simulink model "BEX3_Speed_Contorl_IncrementalEncoders_BLDC_PMSM_2020a"  (R2021b)
settings: Solver=VariableStepAuto  StartTime=0.0  StopTime=1  RelTol=1e-3
(part 1 of 2)
settings Model: Creator=SL_1  LastModifiedBy=SL_1
settings SolverCC: AlgebraicLoopSolver=TrustRegion

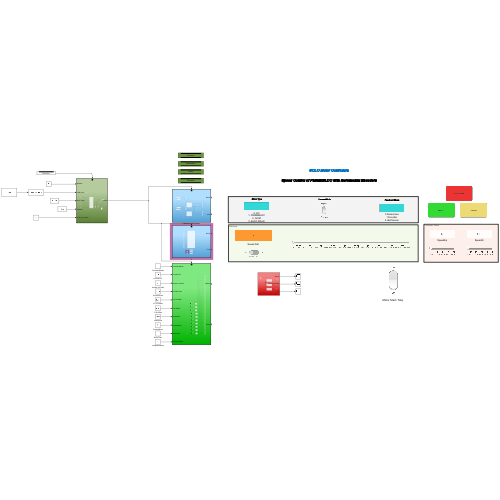
[thumbnail: Simulink's stored preview of the top-level diagram]
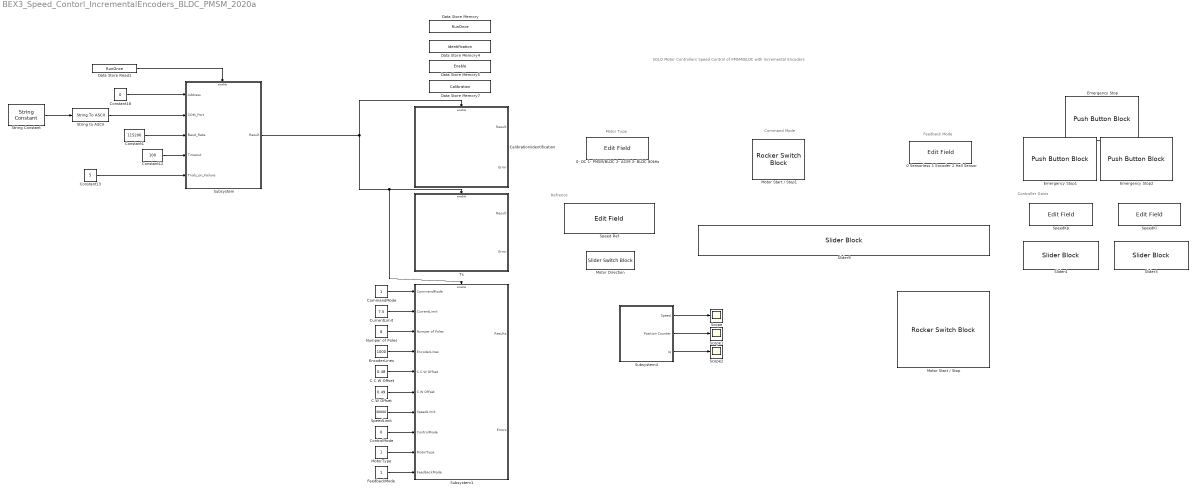
== system BEX3_Speed_Contorl_IncrementalEncoders_BLDC_PMSM_2020a ==
  note: Command Mode
  note: Feedback Mode
  note: Refrence
  note: Controller Gains
  note: SOLO Motor Controllers
      |
      | Speed Control of PMSM/BLDC with Incremental Encoders
  note: Motor Type
  0 Sensorless 1 Encoder 2 Hall Sensor : EditField  LabelPosition=Hide  ShowInitialText=on  Alignment=Center
  "0- DC 1- PMSM/BLDC 2- ACIM 3- BLDC 80kHz " : EditField  LabelPosition=Hide  ShowInitialText=on  Alignment=Center
  C.C.W Offset : Constant  Value=0.48  OutDataTypeStr=single
  C.W Offset : Constant  Value=0.49  OutDataTypeStr=single
  Calibration\Identification : Subsystem
  CommandMode : Constant  OutDataTypeStr=Inherit: Inherit via back propagation  SampleTime=-1
  Constant1 : Constant  Value=115200  OutDataTypeStr=uint32
  Constant12 : Constant  Value=100  OutDataTypeStr=double
  Constant13 : Constant  Value=5  OutDataTypeStr=int32
  Constant18 : Constant  Value=0  OutDataTypeStr=uint8
  ControlMode : Constant  Value=0  OutDataTypeStr=Inherit: Inherit via back propagation
  CurrentLimit : Constant  Value=7.5  OutDataTypeStr=single
  Data Store Memory : DataStoreMemory  DataStoreName=RunOnce  ReadBeforeWriteMsg=warning  WriteAfterWriteMsg=warning  WriteAfterReadMsg=warning  InitialValue=1  ShowAdditionalParam=off  OutDataTypeStr=boolean
  Data Store Memory4 : DataStoreMemory  DataStoreName=Identification  ReadBeforeWriteMsg=warning  WriteAfterWriteMsg=warning  WriteAfterReadMsg=warning  ShowAdditionalParam=off
  Data Store Memory5 : DataStoreMemory  DataStoreName=Enable  ReadBeforeWriteMsg=warning  WriteAfterWriteMsg=warning  WriteAfterReadMsg=warning  ShowAdditionalParam=off
  Data Store Memory7 : DataStoreMemory  DataStoreName=Calibration  ReadBeforeWriteMsg=warning  WriteAfterWriteMsg=warning  WriteAfterReadMsg=warning  ShowAdditionalParam=off
  Data Store Read1 : DataStoreRead  DataStoreName=RunOnce  IndexOptions=Index vector (dialog)  Indices=1  OutputSizes=1
  Emergency Stop : PushButtonBlock  ButtonText=Emergency Stop  OnValue=0  OffValue=1.000000
  Emergency Stop1 : PushButtonBlock  ButtonText=calibration  OffValue=0.000000
  Emergency Stop2 : PushButtonBlock  ButtonText=Identification  OffValue=0.000000
  EncoderLines : Constant  Value=1000  OutDataTypeStr=uint32
  FeedbackMode : Constant  OutDataTypeStr=Inherit: Inherit via back propagation
  Motor Direction : SliderSwitchBlock  LabelPosition=Bottom
      settings: Values={{'CCw', 'Cw'}, [1 0]}
  Motor Start / Stop : RockerSwitchBlock  LabelPosition=Hide
      settings: Values={{'Off', 'On'}, [1 0]}
  Motor Start / Stop1 : RockerSwitchBlock  LabelPosition=Hide
      settings: Values={{'Analog', 'Digital'}, [1 0]}
  MotorType : Constant  OutDataTypeStr=Inherit: Inherit via back propagation
  Numper of Poles : Constant  Value=8  OutDataTypeStr=uint32
  Scope : Scope
  Scope1 : Scope
  Scope2 : Scope
  Slider3 : SliderBlock  LabelPosition=Hide  ScaleMax=5
  Slider4 : SliderBlock  LabelPosition=Hide  ScaleMax=5
  Slider9 : SliderBlock  LabelPosition=Hide  ScaleMax=6000
  Speed Ref : EditField  LabelPosition=Hide  ShowInitialText=on  Alignment=Center
  SpeedKi : EditField  LabelPosition=Hide  ShowInitialText=on  Alignment=Center
  SpeedKp : EditField  LabelPosition=Hide  ShowInitialText=on  Alignment=Center
  SpeedLimit : Constant  Value=30000  OutDataTypeStr=uint32
  String Constant : StringConstant  String="\"COM7\""
  String to ASCII : StringToASCII  OutputVectorSize=5
  Subsystem : Subsystem
  Subsystem1 : Subsystem
  Subsystem4 : Subsystem
  Tx : Subsystem
  wires:
  String Constant/1 -> String to ASCII/1
  Constant18/1 -> Subsystem/1(Address)
  String to ASCII/1 -> Subsystem/2(COM_Port)
  Constant1/1 -> Subsystem/3(Baud_Rate)
  Constant12/1 -> Subsystem/4(Timeout)
  Constant13/1 -> Subsystem/5(Trials_on_Failure)
  FeedbackMode/1 -> Subsystem1/10(FeedbackMode)
  MotorType/1 -> Subsystem1/9(MotorType)
  ControlMode/1 -> Subsystem1/8(ControlMode)
  SpeedLimit/1 -> Subsystem1/7(SpeedLimit)
  C.W Offset/1 -> Subsystem1/6(C.W Offset)
  C.C.W Offset/1 -> Subsystem1/5(C.C.W Offset)
  EncoderLines/1 -> Subsystem1/4(EncoderLines)
  Numper of Poles/1 -> Subsystem1/3(Numper of Poles)
  CurrentLimit/1 -> Subsystem1/2(CurrentLimit)
  CommandMode/1 -> Subsystem1/1(CommandMode)
  Subsystem4/1(Speed) -> Scope/1
  Subsystem4/2(Position Counter) -> Scope1/1
  Subsystem4/3(Iq) -> Scope2/1
  Data Store Read1/1 -> Subsystem/Enable
  Subsystem/1(Result) -> Tx/Enable, Subsystem1/Enable, Calibration\Identification/Enable

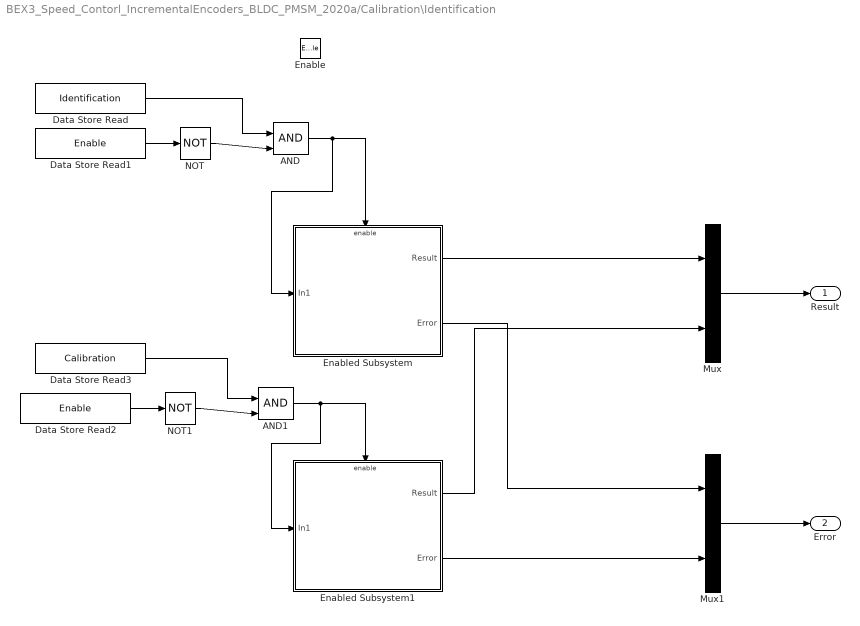
== system BEX3_Speed_Contorl_IncrementalEncoders_BLDC_PMSM_2020a/Calibration\Identification ==
  Enable : EnablePort
  AND : Logic  IconShape=distinctive  AllPortsSameDT=off  OutDataTypeStr=boolean
  AND1 : Logic  IconShape=distinctive  AllPortsSameDT=off  OutDataTypeStr=boolean
  Data Store Read : DataStoreRead  DataStoreName=Identification  IndexOptions=Index vector (dialog)  Indices=1  OutputSizes=1
  Data Store Read1 : DataStoreRead  DataStoreName=Enable  IndexOptions=Index vector (dialog)  Indices=1  OutputSizes=1
  Data Store Read2 : DataStoreRead  DataStoreName=Enable  IndexOptions=Index vector (dialog)  Indices=1  OutputSizes=1
  Data Store Read3 : DataStoreRead  DataStoreName=Calibration  IndexOptions=Index vector (dialog)  Indices=1  OutputSizes=1
  Enabled Subsystem : Subsystem  TreatAsAtomicUnit=on
  Enabled Subsystem1 : Subsystem  TreatAsAtomicUnit=on
  Mux : Mux  Inputs=2
  Mux1 : Mux  Inputs=2
  NOT : Logic  Operator=NOT  IconShape=distinctive  AllPortsSameDT=off  OutDataTypeStr=boolean
  NOT1 : Logic  Operator=NOT  IconShape=distinctive  AllPortsSameDT=off  OutDataTypeStr=boolean
  Result : Outport
  Error : Outport  Port=2
  wires:
  Data Store Read1/1 -> NOT/1
  AND/1 -> Enabled Subsystem/1(In1), Enabled Subsystem/Enable
  NOT/1 -> AND/2
  Data Store Read/1 -> AND/1
  NOT1/1 -> AND1/2
  Data Store Read2/1 -> NOT1/1
  AND1/1 -> Enabled Subsystem1/1(In1), Enabled Subsystem1/Enable
  Data Store Read3/1 -> AND1/1
  Enabled Subsystem/1(Result) -> Mux/1
  Enabled Subsystem/2(Error) -> Mux1/1
  Enabled Subsystem1/2(Error) -> Mux1/2
  Enabled Subsystem1/1(Result) -> Mux/2
  Mux/1 -> Result/1
  Mux1/1 -> Error/1

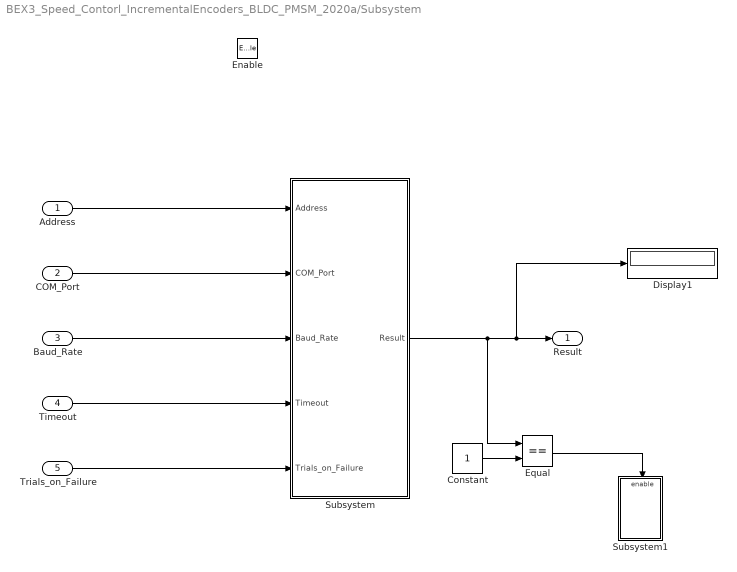
== system BEX3_Speed_Contorl_IncrementalEncoders_BLDC_PMSM_2020a/Subsystem ==
  Address : Inport
  COM_Port : Inport  Port=2
  Baud_Rate : Inport  Port=3
  Timeout : Inport  Port=4
  Trials_on_Failure : Inport  Port=5
  Enable : EnablePort
  Constant : Constant  OutDataTypeStr=Inherit: Inherit via back propagation
  Display1 : Display
  Equal : RelationalOperator  Operator===  OutDataTypeStr=boolean  RndMeth=Simplest
  Subsystem : Subsystem
  Subsystem1 : Subsystem
  Result : Outport
  wires:
  Address/1 -> Subsystem/1(Address)
  COM_Port/1 -> Subsystem/2(COM_Port)
  Baud_Rate/1 -> Subsystem/3(Baud_Rate)
  Timeout/1 -> Subsystem/4(Timeout)
  Trials_on_Failure/1 -> Subsystem/5(Trials_on_Failure)
  Equal/1 -> Subsystem1/Enable
  Subsystem/1(Result) -> Display1/1, Result/1, Equal/1
  Constant/1 -> Equal/2

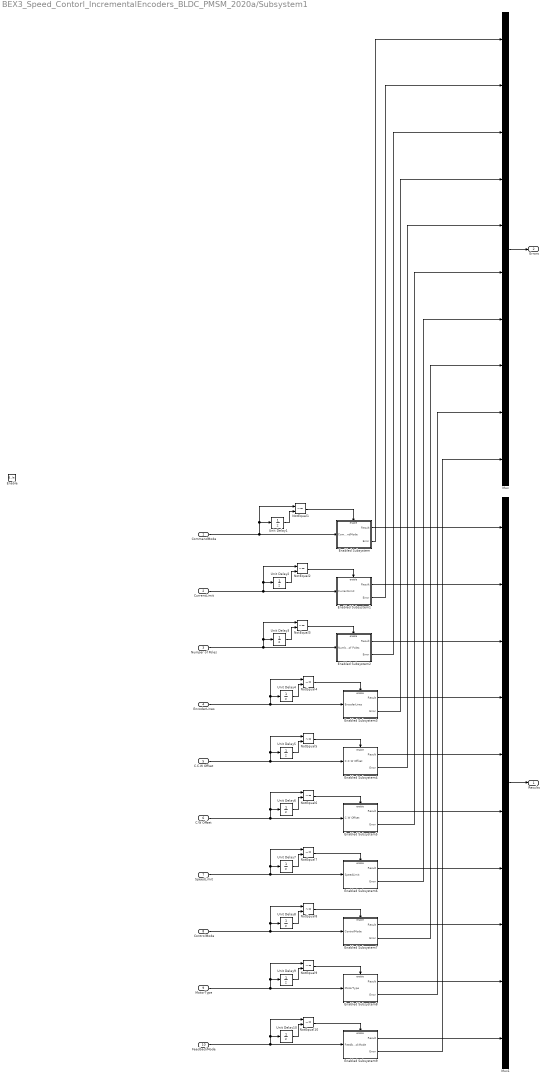
== system BEX3_Speed_Contorl_IncrementalEncoders_BLDC_PMSM_2020a/Subsystem1 ==
  CommandMode : Inport
  CurrentLimit : Inport  Port=2
  Numper of Poles : Inport  Port=3
  EncoderLines : Inport  Port=4
  C.C.W Offset : Inport  Port=5
  C.W Offset : Inport  Port=6
  SpeedLimit : Inport  Port=7
  ControlMode : Inport  Port=8
  MotorType : Inport  Port=9
  FeedbackMode : Inport  Port=10
  Enable : EnablePort
  Enabled Subsystem : Subsystem  TreatAsAtomicUnit=on
  Enabled Subsystem1 : Subsystem  TreatAsAtomicUnit=on
  Enabled Subsystem2 : Subsystem  TreatAsAtomicUnit=on
  Enabled Subsystem3 : Subsystem  TreatAsAtomicUnit=on
  Enabled Subsystem4 : Subsystem  TreatAsAtomicUnit=on
  Enabled Subsystem5 : Subsystem  TreatAsAtomicUnit=on
  Enabled Subsystem6 : Subsystem  TreatAsAtomicUnit=on
  Enabled Subsystem7 : Subsystem  TreatAsAtomicUnit=on
  Enabled Subsystem8 : Subsystem  TreatAsAtomicUnit=on
  Enabled Subsystem9 : Subsystem  TreatAsAtomicUnit=on
  Mux : Mux  Inputs=10
  Mux1 : Mux  Inputs=10
  NotEqual{1..10} (10 alike) : RelationalOperator  Operator=~=  OutDataTypeStr=boolean  RndMeth=Simplest
  Unit Delay{1..10} (10 alike) : UnitDelay  InitialCondition=2.1651  SampleTime=-1  HasFrameUpgradeWarning=on
  Results : Outport
  Errors : Outport  Port=2
  wires:
  Unit Delay1/1 -> NotEqual1/2
  NotEqual1/1 -> Enabled Subsystem/Enable
  NotEqual2/1 -> Enabled Subsystem1/Enable
  CurrentLimit/1 -> NotEqual2/1, Unit Delay2/1, Enabled Subsystem1/1(CurrentLimit)
  Unit Delay2/1 -> NotEqual2/2
  Unit Delay3/1 -> NotEqual3/2
  Numper of Poles/1 -> Enabled Subsystem2/1(Number of Poles), Unit Delay3/1, NotEqual3/1
  NotEqual3/1 -> Enabled Subsystem2/Enable
  NotEqual4/1 -> Enabled Subsystem3/Enable
  EncoderLines/1 -> NotEqual4/1, Unit Delay4/1, Enabled Subsystem3/1(EncoderLines)
  Unit Delay4/1 -> NotEqual4/2
  Unit Delay5/1 -> NotEqual5/2
  C.C.W Offset/1 -> Enabled Subsystem4/1(C.C.W Offset), Unit Delay5/1, NotEqual5/1
  NotEqual5/1 -> Enabled Subsystem4/Enable
  NotEqual6/1 -> Enabled Subsystem5/Enable
  C.W Offset/1 -> NotEqual6/1, Unit Delay6/1, Enabled Subsystem5/1(C.W Offset)
  Unit Delay6/1 -> NotEqual6/2
  Unit Delay7/1 -> NotEqual7/2
  SpeedLimit/1 -> Enabled Subsystem6/1(SpeedLimit), Unit Delay7/1, NotEqual7/1
  NotEqual7/1 -> Enabled Subsystem6/Enable
  NotEqual8/1 -> Enabled Subsystem7/Enable
  ControlMode/1 -> NotEqual8/1, Unit Delay8/1, Enabled Subsystem7/1(ControlMode)
  Unit Delay8/1 -> NotEqual8/2
  Unit Delay9/1 -> NotEqual9/2
  MotorType/1 -> Enabled Subsystem8/1(MotorType), Unit Delay9/1, NotEqual9/1
  NotEqual9/1 -> Enabled Subsystem8/Enable
  NotEqual10/1 -> Enabled Subsystem9/Enable
  FeedbackMode/1 -> NotEqual10/1, Unit Delay10/1, Enabled Subsystem9/1(FeedbackMode)
  Unit Delay10/1 -> NotEqual10/2
  CommandMode/1 -> Enabled Subsystem/1(CommandMode), NotEqual1/1, Unit Delay1/1
  Enabled Subsystem9/2(Error) -> Mux/10
  Enabled Subsystem8/2(Error) -> Mux/9
  Enabled Subsystem7/2(Error) -> Mux/8
  Enabled Subsystem6/2(Error) -> Mux/7
  Enabled Subsystem5/2(Error) -> Mux/6
  Enabled Subsystem4/2(Error) -> Mux/5
  Enabled Subsystem3/2(Error) -> Mux/4
  Enabled Subsystem2/2(Error) -> Mux/3
  Enabled Subsystem1/2(Error) -> Mux/2
  Enabled Subsystem/2(Error) -> Mux/1
  Enabled Subsystem/1(Result) -> Mux1/1
  Enabled Subsystem1/1(Result) -> Mux1/2
  Enabled Subsystem2/1(Result) -> Mux1/3
  Enabled Subsystem3/1(Result) -> Mux1/4
  Enabled Subsystem5/1(Result) -> Mux1/6
  Enabled Subsystem7/1(Result) -> Mux1/8
  Enabled Subsystem6/1(Result) -> Mux1/7
  Enabled Subsystem8/1(Result) -> Mux1/9
  Enabled Subsystem9/1(Result) -> Mux1/10
  Enabled Subsystem4/1(Result) -> Mux1/5
  Mux1/1 -> Results/1
  Mux/1 -> Errors/1

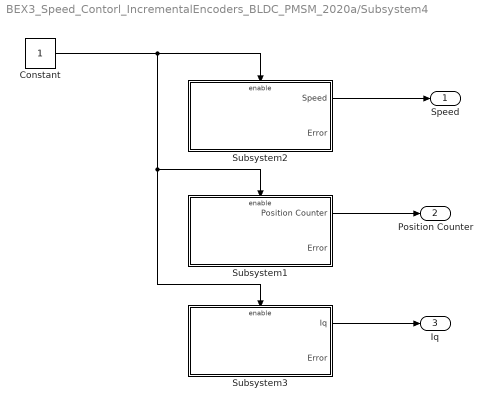
== system BEX3_Speed_Contorl_IncrementalEncoders_BLDC_PMSM_2020a/Subsystem4 ==
  Constant : Constant  SampleTime=1e-3
  Subsystem1 : Subsystem
  Subsystem2 : Subsystem
  Subsystem3 : Subsystem
  Speed : Outport
  Position Counter : Outport  Port=2
  Iq : Outport  Port=3
  wires:
  Constant/1 -> Subsystem1/Enable, Subsystem3/Enable, Subsystem2/Enable
  Subsystem2/1(Speed) -> Speed/1
  Subsystem1/1(Position Counter) -> Position Counter/1
  Subsystem3/1(Iq) -> Iq/1

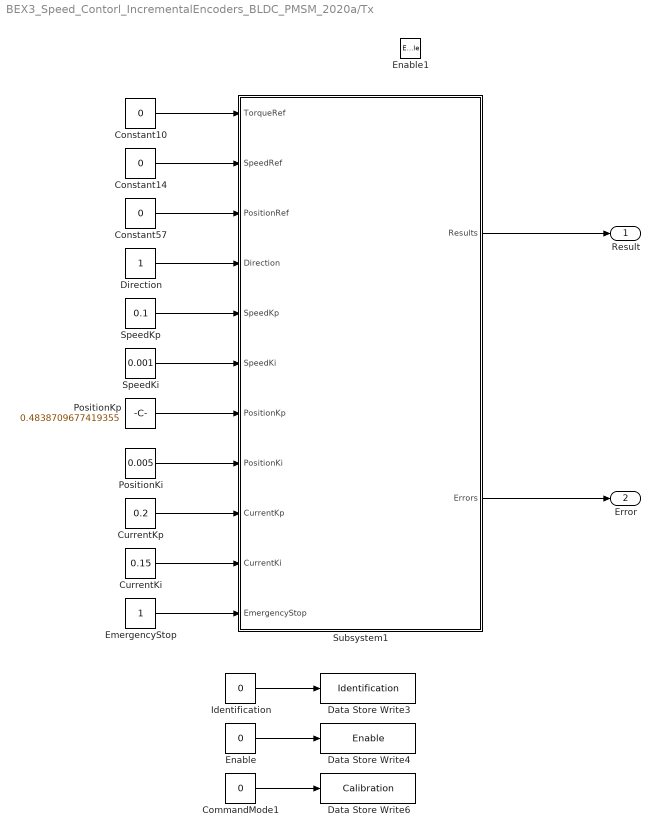
== system BEX3_Speed_Contorl_IncrementalEncoders_BLDC_PMSM_2020a/Tx ==
  Enable1 : EnablePort
  CommandMode1 : Constant  Value=0  OutDataTypeStr=Inherit: Inherit via back propagation
  Constant10 : Constant  Value=0  OutDataTypeStr=Inherit: Inherit via back propagation
  Constant14 : Constant  Value=0  OutDataTypeStr=Inherit: Inherit via back propagation
  Constant57 : Constant  Value=0  OutDataTypeStr=Inherit: Inherit via back propagation
  CurrentKi : Constant  Value=0.15  OutDataTypeStr=Inherit: Inherit via back propagation
  CurrentKp : Constant  Value=0.2  OutDataTypeStr=Inherit: Inherit via back propagation
  Data Store Write3 : DataStoreWrite  DataStoreName=Identification  IndexOptions=Index vector (dialog)  Indices=1  OutputSizes=1
  Data Store Write4 : DataStoreWrite  DataStoreName=Enable  IndexOptions=Index vector (dialog)  Indices=1  OutputSizes=1
  Data Store Write6 : DataStoreWrite  DataStoreName=Calibration  IndexOptions=Index vector (dialog)  Indices=1  OutputSizes=1
  Direction : Constant  OutDataTypeStr=Inherit: Inherit via back propagation
  EmergencyStop : Constant  OutDataTypeStr=boolean
  Enable : Constant  Value=0  OutDataTypeStr=Inherit: Inherit via back propagation
  Identification : Constant  Value=0  OutDataTypeStr=Inherit: Inherit via back propagation
  PositionKi : Constant  Value=0.005  OutDataTypeStr=Inherit: Inherit via back propagation
  PositionKp : Constant  Value=0.4838709677419355  OutDataTypeStr=Inherit: Inherit via back propagation
  SpeedKi : Constant  Value=0.001  OutDataTypeStr=Inherit: Inherit via back propagation
  SpeedKp : Constant  Value=0.1  OutDataTypeStr=Inherit: Inherit via back propagation
  Subsystem1 : Subsystem
  Result : Outport
  Error : Outport  Port=2
  wires:
  Direction/1 -> Subsystem1/4(Direction)
  Constant10/1 -> Subsystem1/1(TorqueRef)
  Constant14/1 -> Subsystem1/2(SpeedRef)
  Constant57/1 -> Subsystem1/3(PositionRef)
  CurrentKi/1 -> Subsystem1/10(CurrentKi)
  CurrentKp/1 -> Subsystem1/9(CurrentKp)
  PositionKi/1 -> Subsystem1/8(PositionKi)
  PositionKp/1 -> Subsystem1/7(PositionKp)
  SpeedKi/1 -> Subsystem1/6(SpeedKi)
  SpeedKp/1 -> Subsystem1/5(SpeedKp)
  Identification/1 -> Data Store Write3/1
  Enable/1 -> Data Store Write4/1
  EmergencyStop/1 -> Subsystem1/11(EmergencyStop)
  CommandMode1/1 -> Data Store Write6/1
  Subsystem1/1(Results) -> Result/1
  Subsystem1/2(Errors) -> Error/1

== system BEX3_Speed_Contorl_IncrementalEncoders_BLDC_PMSM_2020a/Calibration\Identification/Enabled Subsystem ==
  In1 : Inport
  Enable : EnablePort
  Constant21 : Constant  Value=0  OutDataTypeStr=uint8
  MotorParameterIdentification : Subsystem
  Result : Outport
  Error : Outport  Port=2
  wires:
  In1/1 -> MotorParameterIdentification/2(Value)
  Constant21/1 -> MotorParameterIdentification/1(Address)
  MotorParameterIdentification/1(Result) -> Result/1
  MotorParameterIdentification/2(Error) -> Error/1

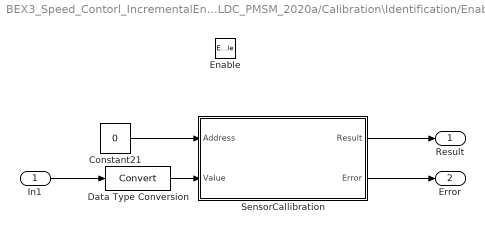
== system BEX3_Speed_Contorl_IncrementalEncoders_BLDC_PMSM_2020a/Calibration\Identification/Enabled Subsystem1 ==
  In1 : Inport
  Enable : EnablePort
  Constant21 : Constant  Value=0  OutDataTypeStr=uint8
  Data Type Conversion : DataTypeConversion
  SensorCallibration : Subsystem
  Result : Outport
  Error : Outport  Port=2
  wires:
  Constant21/1 -> SensorCallibration/1(Address)
  In1/1 -> Data Type Conversion/1
  Data Type Conversion/1 -> SensorCallibration/2(Value)
  SensorCallibration/1(Result) -> Result/1
  SensorCallibration/2(Error) -> Error/1

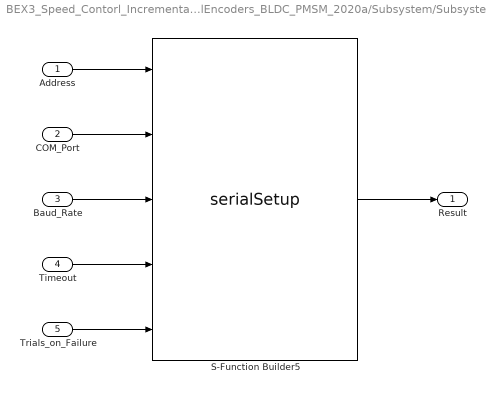
== system BEX3_Speed_Contorl_IncrementalEncoders_BLDC_PMSM_2020a/Subsystem/Subsystem ==
  Address : Inport
  COM_Port : Inport  Port=2
  Baud_Rate : Inport  Port=3
  Timeout : Inport  Port=4
  Trials_on_Failure : Inport  Port=5
  S-Function Builder5 : S-Function  Priority=1  FunctionName=serialSetup  SFunctionModules=serialSetup_wrapper  SFunctionDeploymentMode=off  EnableBusSupport=off  mask(S-Function Builder){}
      mask help: Simulink:masks:SFunctionBuilder_MD
      mask init:
      | val = [[.9  0.75 0.75 1 1 .9 .9 1]',[1 1 0.75 0.75 .9 .9 1 .9]'];try , sys = get_param(gcb,'SfunBuilderFcnName');if isempty(sys), sys = get_param(gcb,'FunctionName'); end,catch, sys = get_param(gcb,'FunctionName'); end
      settings: CopyFcn=set_param(gcbh,'LinkStatus','none')  OpenFcn=sfunctionwizard(gcbh)
      mask Display: plot(val(:,1),val(:,2)),disp(sys),port_label('input',1,'Address'),port_label('input',2,'COM_Port'),port_label('input',3,'Baud_Rate'),port_label('input',4,'Timeout'),port_label('input',5,'Trials_on_Failure'),port_label('output',1,'Result')
  Result : Outport
  wires:
  S-Function Builder5/1 -> Result/1
  COM_Port/1 -> S-Function Builder5/2
  Address/1 -> S-Function Builder5/1
  Timeout/1 -> S-Function Builder5/4
  Baud_Rate/1 -> S-Function Builder5/3
  Trials_on_Failure/1 -> S-Function Builder5/5

== system BEX3_Speed_Contorl_IncrementalEncoders_BLDC_PMSM_2020a/Subsystem/Subsystem1 ==
  Enable : EnablePort
  Constant1 : Constant  Value=0  OutDataTypeStr=Inherit: Inherit via back propagation
  Data Store Write : DataStoreWrite  DataStoreName=RunOnce  IndexOptions=Index vector (dialog)  Indices=1  OutputSizes=1
  wires:
  Constant1/1 -> Data Store Write/1

== system BEX3_Speed_Contorl_IncrementalEncoders_BLDC_PMSM_2020a/Subsystem1/Enabled Subsystem ==
  CommandMode : Inport
  Enable : EnablePort
  Constant6 : Constant  Value=0  OutDataTypeStr=Inherit: Inherit via back propagation
  SetCommandMode : Subsystem
  Result : Outport
  Error : Outport  Port=2
  wires:
  Constant6/1 -> SetCommandMode/1(Address)
  CommandMode/1 -> SetCommandMode/2(Value)
  SetCommandMode/1(Result) -> Result/1
  SetCommandMode/2(Error) -> Error/1

== system BEX3_Speed_Contorl_IncrementalEncoders_BLDC_PMSM_2020a/Subsystem1/Enabled Subsystem1 ==
  CurrentLimit : Inport
  Enable : EnablePort
  Constant6 : Constant  Value=0  OutDataTypeStr=uint8
  SetCurrentLimit : Subsystem
  Result : Outport
  Error : Outport  Port=2
  wires:
  Constant6/1 -> SetCurrentLimit/1(Address)
  CurrentLimit/1 -> SetCurrentLimit/2(Value)
  SetCurrentLimit/2(Error) -> Error/1
  SetCurrentLimit/1(Result) -> Result/1

== system BEX3_Speed_Contorl_IncrementalEncoders_BLDC_PMSM_2020a/Subsystem1/Enabled Subsystem2 ==
  Number of Poles : Inport
  Enable : EnablePort
  Constant6 : Constant  Value=0  OutDataTypeStr=uint8
  SetMotorPoleCounts : Subsystem
  Result : Outport
  Error : Outport  Port=2
  wires:
  Number of Poles/1 -> SetMotorPoleCounts/2(Value)
  Constant6/1 -> SetMotorPoleCounts/1(Address)
  SetMotorPoleCounts/2(Error) -> Error/1
  SetMotorPoleCounts/1(Result) -> Result/1

== system BEX3_Speed_Contorl_IncrementalEncoders_BLDC_PMSM_2020a/Subsystem1/Enabled Subsystem3 ==
  EncoderLines : Inport
  Enable : EnablePort
  Constant6 : Constant  Value=0  OutDataTypeStr=uint8
  SetEncoderLines : Subsystem
  Result : Outport
  Error : Outport  Port=2
  wires:
  Constant6/1 -> SetEncoderLines/1(Address)
  EncoderLines/1 -> SetEncoderLines/2(Value)
  SetEncoderLines/2(Error) -> Error/1
  SetEncoderLines/1(Result) -> Result/1

== system BEX3_Speed_Contorl_IncrementalEncoders_BLDC_PMSM_2020a/Subsystem1/Enabled Subsystem4 ==
  C.C.W Offset : Inport
  Enable : EnablePort
  Constant6 : Constant  Value=0  OutDataTypeStr=uint8
  SetEncoderHallCcwOffset : Subsystem
  Result : Outport
  Error : Outport  Port=2
  wires:
  C.C.W Offset/1 -> SetEncoderHallCcwOffset/2(Value)
  Constant6/1 -> SetEncoderHallCcwOffset/1(Address)
  SetEncoderHallCcwOffset/2(Error) -> Error/1
  SetEncoderHallCcwOffset/1(Result) -> Result/1

== system BEX3_Speed_Contorl_IncrementalEncoders_BLDC_PMSM_2020a/Subsystem1/Enabled Subsystem5 ==
  C.W Offset : Inport
  Enable : EnablePort
  Constant6 : Constant  Value=0  OutDataTypeStr=uint8
  SetEncoderHallCwOffset : Subsystem
  Result : Outport
  Error : Outport  Port=2
  wires:
  Constant6/1 -> SetEncoderHallCwOffset/1(Address)
  C.W Offset/1 -> SetEncoderHallCwOffset/2(Value)
  SetEncoderHallCwOffset/2(Error) -> Error/1
  SetEncoderHallCwOffset/1(Result) -> Result/1

== system BEX3_Speed_Contorl_IncrementalEncoders_BLDC_PMSM_2020a/Subsystem1/Enabled Subsystem6 ==
  SpeedLimit : Inport
  Enable : EnablePort
  Constant6 : Constant  Value=0  OutDataTypeStr=uint8
  SetSpeedLimit : Subsystem
  Result : Outport
  Error : Outport  Port=2
  wires:
  SpeedLimit/1 -> SetSpeedLimit/2(Value)
  Constant6/1 -> SetSpeedLimit/1(Address)
  SetSpeedLimit/2(Error) -> Error/1
  SetSpeedLimit/1(Result) -> Result/1

== system BEX3_Speed_Contorl_IncrementalEncoders_BLDC_PMSM_2020a/Subsystem1/Enabled Subsystem7 ==
  ControlMode : Inport
  Enable : EnablePort
  Constant6 : Constant  Value=0  OutDataTypeStr=uint8
  SetControlMode : Subsystem
  Result : Outport
  Error : Outport  Port=2
  wires:
  Constant6/1 -> SetControlMode/1(Address)
  ControlMode/1 -> SetControlMode/2(Value)
  SetControlMode/2(Error) -> Error/1
  SetControlMode/1(Result) -> Result/1

== system BEX3_Speed_Contorl_IncrementalEncoders_BLDC_PMSM_2020a/Subsystem1/Enabled Subsystem8 ==
  MotorType : Inport
  Enable : EnablePort
  Constant6 : Constant  Value=0  OutDataTypeStr=uint8
  SetMotorType : Subsystem
  Result : Outport
  Error : Outport  Port=2
  wires:
  MotorType/1 -> SetMotorType/2(Value)
  Constant6/1 -> SetMotorType/1(Address)
  SetMotorType/2(Error) -> Error/1
  SetMotorType/1(Result) -> Result/1

== system BEX3_Speed_Contorl_IncrementalEncoders_BLDC_PMSM_2020a/Subsystem1/Enabled Subsystem9 ==
  FeedbackMode : Inport
  Enable : EnablePort
  Constant6 : Constant  Value=0  OutDataTypeStr=uint8
  SetFeedBackControlMode : Subsystem
  Result : Outport
  Error : Outport  Port=2
  wires:
  Constant6/1 -> SetFeedBackControlMode/1(Address)
  FeedbackMode/1 -> SetFeedBackControlMode/2(Value)
  SetFeedBackControlMode/2(Error) -> Error/1
  SetFeedBackControlMode/1(Result) -> Result/1

== system BEX3_Speed_Contorl_IncrementalEncoders_BLDC_PMSM_2020a/Subsystem4/Subsystem1 ==
  Enable : EnablePort
  Constant120 : Constant  Value=0  OutDataTypeStr=uint8
  GetPositionCountsFeedback : Subsystem
  Position Counter : Outport
  Error : Outport  Port=2
  wires:
  Constant120/1 -> GetPositionCountsFeedback/1(Address)
  GetPositionCountsFeedback/1(Result) -> Position Counter/1
  GetPositionCountsFeedback/2(Error) -> Error/1

== system BEX3_Speed_Contorl_IncrementalEncoders_BLDC_PMSM_2020a/Subsystem4/Subsystem2 ==
  Enable : EnablePort
  Constant120 : Constant  Value=0  OutDataTypeStr=uint8
  GetSpeedFeedback : Subsystem
  Speed : Outport
  Error : Outport  Port=2
  wires:
  GetSpeedFeedback/1(Result) -> Speed/1
  Constant120/1 -> GetSpeedFeedback/1(Address)
  GetSpeedFeedback/2(Error) -> Error/1

== system BEX3_Speed_Contorl_IncrementalEncoders_BLDC_PMSM_2020a/Subsystem4/Subsystem3 ==
  Enable : EnablePort
  Constant120 : Constant  Value=0  OutDataTypeStr=uint8
  GetQuadratureCurrentIqFeedback : Subsystem
  Iq : Outport
  Error : Outport  Port=2
  wires:
  GetQuadratureCurrentIqFeedback/2(Error) -> Error/1
  GetQuadratureCurrentIqFeedback/1(Result) -> Iq/1
  Constant120/1 -> GetQuadratureCurrentIqFeedback/1(Address)

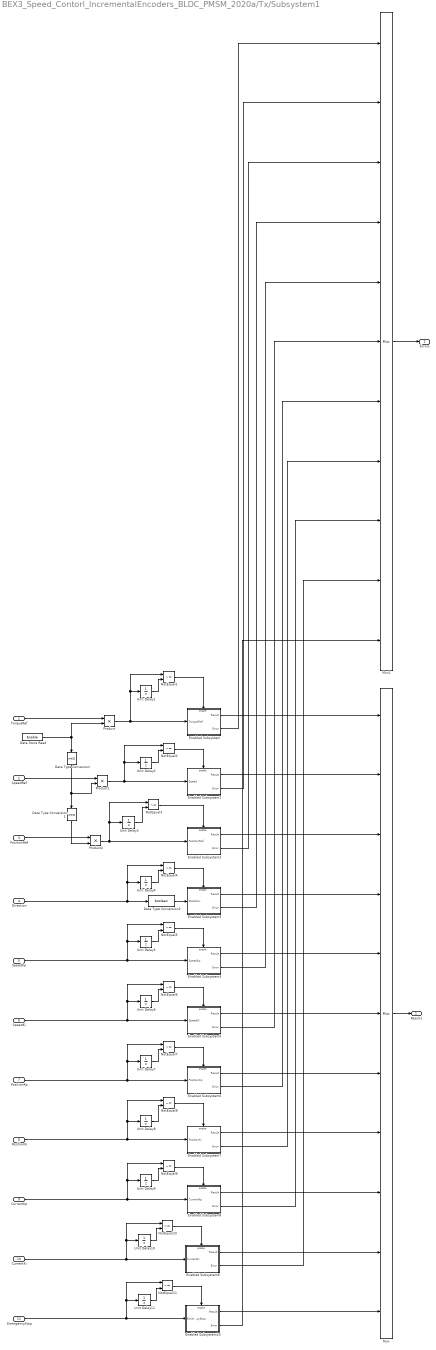
== system BEX3_Speed_Contorl_IncrementalEncoders_BLDC_PMSM_2020a/Tx/Subsystem1 ==
  TorqueRef : Inport
  SpeedRef : Inport  Port=2
  PositionRef : Inport  Port=3
  Direction : Inport  Port=4
  SpeedKp : Inport  Port=5
  SpeedKi : Inport  Port=6
  PositionKp : Inport  Port=7
  PositionKi : Inport  Port=8
  CurrentKp : Inport  Port=9
  CurrentKi : Inport  Port=10
  EmergencyStop : Inport  Port=11
  Data Store Read : DataStoreRead  DataStoreName=Enable  IndexOptions=Index vector (dialog)  Indices=1  OutputSizes=1
  Data Type Conversion : DataTypeConversion  OutDataTypeStr=uint32
  Data Type Conversion1 : DataTypeConversion  OutDataTypeStr=uint32
  Data Type Conversion2 : DataTypeConversion  OutDataTypeStr=boolean
  Enabled Subsystem : Subsystem  TreatAsAtomicUnit=on
  Enabled Subsystem1 : Subsystem  TreatAsAtomicUnit=on
  Enabled Subsystem10 : Subsystem  TreatAsAtomicUnit=on
  Enabled Subsystem2 : Subsystem  TreatAsAtomicUnit=on
  Enabled Subsystem3 : Subsystem  TreatAsAtomicUnit=on
  Enabled Subsystem4 : Subsystem  TreatAsAtomicUnit=on
  Enabled Subsystem5 : Subsystem  TreatAsAtomicUnit=on
  Enabled Subsystem6 : Subsystem  TreatAsAtomicUnit=on
  Enabled Subsystem7 : Subsystem  TreatAsAtomicUnit=on
  Enabled Subsystem8 : Subsystem  TreatAsAtomicUnit=on
  Enabled Subsystem9 : Subsystem  TreatAsAtomicUnit=on
  Mux : Mux  Inputs=11
  Mux1 : Mux  Inputs=11
  NotEqual{1..11} (11 alike) : RelationalOperator  Operator=~=  OutDataTypeStr=boolean  RndMeth=Simplest
  Product : Product
  Product1 : Product  OutDataTypeStr=Inherit: Inherit via back propagation
  Product2 : Product  OutDataTypeStr=Inherit: Inherit via back propagation
  Unit Delay{1..11} (11 alike) : UnitDelay  InitialCondition=2.1651  SampleTime=-1  HasFrameUpgradeWarning=on
  Results : Outport
  Errors : Outport  Port=2
  wires:
  TorqueRef/1 -> Product/1
  Unit Delay1/1 -> NotEqual1/2
  NotEqual1/1 -> Enabled Subsystem/Enable
  Data Store Read/1 -> Data Type Conversion/1, Product/2
  Product/1 -> Enabled Subsystem/1(TorqueRef), Unit Delay1/1, NotEqual1/1
  NotEqual2/1 -> Enabled Subsystem1/Enable
  Unit Delay2/1 -> NotEqual2/2
  SpeedRef/1 -> Product1/1
  Product1/1 -> Unit Delay2/1, NotEqual2/1, Enabled Subsystem1/1(Speed)
  PositionRef/1 -> Product2/1
  Unit Delay3/1 -> NotEqual3/2
  NotEqual3/1 -> Enabled Subsystem2/Enable
  Direction/1 -> NotEqual4/1, Unit Delay4/1, Data Type Conversion2/1
  Unit Delay4/1 -> NotEqual4/2
  NotEqual4/1 -> Enabled Subsystem3/Enable
  NotEqual5/1 -> Enabled Subsystem4/Enable
  Unit Delay5/1 -> NotEqual5/2
  SpeedKp/1 -> Enabled Subsystem4/1(SpeedKp), Unit Delay5/1, NotEqual5/1
  SpeedKi/1 -> Enabled Subsystem5/1(SpeedKi), NotEqual6/1, Unit Delay6/1
  Unit Delay6/1 -> NotEqual6/2
  NotEqual6/1 -> Enabled Subsystem5/Enable
  NotEqual7/1 -> Enabled Subsystem6/Enable
  Unit Delay7/1 -> NotEqual7/2
  PositionKp/1 -> Enabled Subsystem6/1(PositionKp), Unit Delay7/1, NotEqual7/1
  PositionKi/1 -> Enabled Subsystem7/1(PositionKi), NotEqual8/1, Unit Delay8/1
  Unit Delay8/1 -> NotEqual8/2
  NotEqual8/1 -> Enabled Subsystem7/Enable
  NotEqual9/1 -> Enabled Subsystem8/Enable
  Unit Delay9/1 -> NotEqual9/2
  CurrentKp/1 -> Enabled Subsystem8/1(CurrentKp), Unit Delay9/1, NotEqual9/1
  CurrentKi/1 -> Enabled Subsystem9/1(CurrentKi), NotEqual10/1, Unit Delay10/1
  Unit Delay10/1 -> NotEqual10/2
  NotEqual10/1 -> Enabled Subsystem9/Enable
  NotEqual11/1 -> Enabled Subsystem10/Enable
  Unit Delay11/1 -> NotEqual11/2
  EmergencyStop/1 -> Unit Delay11/1, NotEqual11/1, Enabled Subsystem10/1(EmergencyStop)
  Data Type Conversion/1 -> Product1/2, Data Type Conversion1/1
  Data Type Conversion1/1 -> Product2/2
  Product2/1 -> NotEqual3/1, Unit Delay3/1, Enabled Subsystem2/1(PositionRef)
  Data Type Conversion2/1 -> Enabled Subsystem3/1(Direction)
  Enabled Subsystem/1(Result) -> Mux/1
  Enabled Subsystem10/1(Result) -> Mux/11
  Enabled Subsystem9/1(Result) -> Mux/10
  Enabled Subsystem8/1(Result) -> Mux/9
  Enabled Subsystem7/1(Result) -> Mux/8
  Enabled Subsystem6/1(Result) -> Mux/7
  Enabled Subsystem5/1(Result) -> Mux/6
  Enabled Subsystem4/1(Result) -> Mux/5
  Enabled Subsystem3/1(Result) -> Mux/4
  Enabled Subsystem2/1(Result) -> Mux/3
  Enabled Subsystem1/1(Result) -> Mux/2
  Mux/1 -> Results/1
  Enabled Subsystem/2(Error) -> Mux1/1
  Enabled Subsystem1/2(Error) -> Mux1/2
  Enabled Subsystem2/2(Error) -> Mux1/3
  Enabled Subsystem3/2(Error) -> Mux1/4
  Enabled Subsystem4/2(Error) -> Mux1/5
  Enabled Subsystem5/2(Error) -> Mux1/6
  Enabled Subsystem6/2(Error) -> Mux1/7
  Enabled Subsystem7/2(Error) -> Mux1/8
  Enabled Subsystem8/2(Error) -> Mux1/9
  Enabled Subsystem9/2(Error) -> Mux1/10
  Enabled Subsystem10/2(Error) -> Mux1/11
  Mux1/1 -> Errors/1

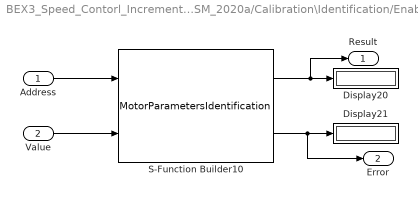
== system BEX3_Speed_Contorl_IncrementalEncoders_BLDC_PMSM_2020a/Calibration\Identification/Enabled Subsystem/MotorParameterIdentification ==
  Address : Inport
  Value : Inport  Port=2
  Display20 : Display
      settings: Format=decimal (Stored Integer)
  Display21 : Display
      settings: Format=decimal (Stored Integer)
  S-Function Builder10 : S-Function  Priority=2  FunctionName=MotorParametersIdentification  SFunctionModules=MotorParametersIdentification_wrapper  SFunctionDeploymentMode=off  EnableBusSupport=off  mask(S-Function Builder){}
      mask help: Simulink:masks:SFunctionBuilder_MD
      mask init: same as BEX3_Speed_Contorl_IncrementalEncoders_BLDC_PMSM_2020a/Subsystem/Subsystem/S-Function Builder5
      settings: CopyFcn=set_param(gcbh,'LinkStatus','none')  OpenFcn=sfunctionwizard(gcbh)
      mask Display:
      | plot(val(:,1),val(:,2))
      | disp(sys)
      | port_label('input',1,'Address')
      | port_label('input',2,'Value')
      | port_label('output',1,'Result')
      | port_label('output',2,'Error')
  Result : Outport
  Error : Outport  Port=2
  wires:
  S-Function Builder10/2 -> Error/1, Display21/1
  S-Function Builder10/1 -> Result/1, Display20/1
  Value/1 -> S-Function Builder10/2
  Address/1 -> S-Function Builder10/1

== system BEX3_Speed_Contorl_IncrementalEncoders_BLDC_PMSM_2020a/Calibration\Identification/Enabled Subsystem1/SensorCallibration ==
  Address : Inport
  Value : Inport  Port=2
  S-Function Builder41 : S-Function  Priority=2  FunctionName=SensorCalibration  SFunctionModules=SensorCalibration_wrapper  SFunctionDeploymentMode=off  EnableBusSupport=off  mask(S-Function Builder){}
      mask help: Simulink:masks:SFunctionBuilder_MD
      mask init: same as BEX3_Speed_Contorl_IncrementalEncoders_BLDC_PMSM_2020a/Subsystem/Subsystem/S-Function Builder5
      settings: CopyFcn=set_param(gcbh,'LinkStatus','none')  OpenFcn=sfunctionwizard(gcbh)
      mask Display:
      | plot(val(:,1),val(:,2))
      | disp(sys)
      | port_label('input',1,'Address')
      | port_label('input',2,'Value')
      | port_label('output',1,'Result')
      | port_label('output',2,'Error')
  Result : Outport
  Error : Outport  Port=2
  wires:
  Value/1 -> S-Function Builder41/2
  S-Function Builder41/1 -> Result/1
  Address/1 -> S-Function Builder41/1
  S-Function Builder41/2 -> Error/1

== system BEX3_Speed_Contorl_IncrementalEncoders_BLDC_PMSM_2020a/Subsystem1/Enabled Subsystem/SetCommandMode ==
  Address : Inport  OutDataTypeStr=uint8  LockScale=on
  Value : Inport  Port=2  OutDataTypeStr=boolean  LockScale=on
  S-Function Builder2 : S-Function  Priority=2  FunctionName=SetCommandMode  SFunctionModules=SetCommandMode_wrapper  SFunctionDeploymentMode=off  EnableBusSupport=off  mask(S-Function Builder){}
      mask help: Simulink:masks:SFunctionBuilder_MD
      mask init: same as BEX3_Speed_Contorl_IncrementalEncoders_BLDC_PMSM_2020a/Subsystem/Subsystem/S-Function Builder5
      settings: CopyFcn=set_param(gcbh,'LinkStatus','none')  OpenFcn=sfunctionwizard(gcbh)
      mask Display: plot(val(:,1),val(:,2)),disp(sys),port_label('input',1,'Address'),port_label('input',2,'Value'),port_label('output',1,'Result'),port_label('output',2,'Error')
  Result : Outport  OutDataTypeStr=boolean
  Error : Outport  Port=2
  wires:
  S-Function Builder2/1 -> Result/1
  S-Function Builder2/2 -> Error/1
  Address/1 -> S-Function Builder2/1
  Value/1 -> S-Function Builder2/2

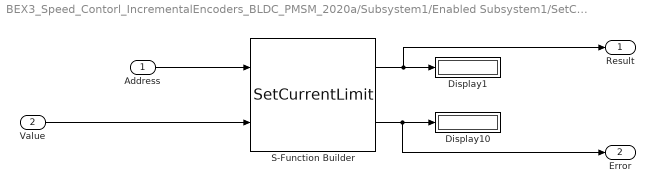
== system BEX3_Speed_Contorl_IncrementalEncoders_BLDC_PMSM_2020a/Subsystem1/Enabled Subsystem1/SetCurrentLimit ==
  Address : Inport  Tag=Address  LockScale=on
  Value : Inport  Port=2  LockScale=on
  Display1 : Display
      settings: Format=decimal (Stored Integer)
  Display10 : Display
      settings: Format=decimal (Stored Integer)
  S-Function Builder : S-Function  Priority=2  FunctionName=SetCurrentLimit  SFunctionModules=SetCurrentLimit_wrapper  SFunctionDeploymentMode=off  EnableBusSupport=off  mask(S-Function Builder){}
      mask help: Simulink:masks:SFunctionBuilder_MD
      mask init: same as BEX3_Speed_Contorl_IncrementalEncoders_BLDC_PMSM_2020a/Subsystem/Subsystem/S-Function Builder5
      settings: CopyFcn=set_param(gcbh,'LinkStatus','none')  OpenFcn=sfunctionwizard(gcbh)
      mask Display: plot(val(:,1),val(:,2)),disp(sys),port_label('input',1,'Address'),port_label('input',2,'Value'),port_label('output',1,'Result'),port_label('output',2,'Error')
  Result : Outport  OutDataTypeStr=boolean
  Error : Outport  Port=2  OutDataTypeStr=int32
  wires:
  Value/1 -> S-Function Builder/2
  S-Function Builder/2 -> Error/1, Display10/1
  S-Function Builder/1 -> Result/1, Display1/1
  Address/1 -> S-Function Builder/1

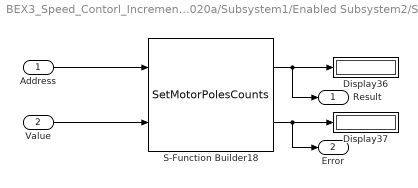
== system BEX3_Speed_Contorl_IncrementalEncoders_BLDC_PMSM_2020a/Subsystem1/Enabled Subsystem2/SetMotorPoleCounts ==
  Address : Inport
  Value : Inport  Port=2
  Display36 : Display
      settings: Format=decimal (Stored Integer)
  Display37 : Display
      settings: Format=decimal (Stored Integer)
  S-Function Builder18 : S-Function  Priority=2  FunctionName=SetMotorPolesCounts  SFunctionModules=SetMotorPolesCounts_wrapper  SFunctionDeploymentMode=off  EnableBusSupport=off  mask(S-Function Builder){}
      mask help: Simulink:masks:SFunctionBuilder_MD
      mask init: same as BEX3_Speed_Contorl_IncrementalEncoders_BLDC_PMSM_2020a/Subsystem/Subsystem/S-Function Builder5
      settings: CopyFcn=set_param(gcbh,'LinkStatus','none')  OpenFcn=sfunctionwizard(gcbh)
      mask Display:
      | plot(val(:,1),val(:,2))
      | disp(sys)
      | port_label('input',1,'Address')
      | port_label('input',2,'Value')
      | port_label('output',1,'Result')
      | port_label('output',2,'Error')
  Result : Outport
  Error : Outport  Port=2
  wires:
  S-Function Builder18/1 -> Result/1, Display36/1
  Value/1 -> S-Function Builder18/2
  S-Function Builder18/2 -> Error/1, Display37/1
  Address/1 -> S-Function Builder18/1

== system BEX3_Speed_Contorl_IncrementalEncoders_BLDC_PMSM_2020a/Subsystem1/Enabled Subsystem3/SetEncoderLines ==
  Address : Inport
  Value : Inport  Port=2
  Display38 : Display
      settings: Format=decimal (Stored Integer)
  Display39 : Display
      settings: Format=decimal (Stored Integer)
  S-Function Builder19 : S-Function  Priority=2  FunctionName=SetIncrementalEncoderLines  SFunctionModules=SetIncrementalEncoderLines_wrapper  SFunctionDeploymentMode=off  EnableBusSupport=off  mask(S-Function Builder){}
      mask help: Simulink:masks:SFunctionBuilder_MD
      mask init: same as BEX3_Speed_Contorl_IncrementalEncoders_BLDC_PMSM_2020a/Subsystem/Subsystem/S-Function Builder5
      settings: CopyFcn=set_param(gcbh,'LinkStatus','none')  OpenFcn=sfunctionwizard(gcbh)
      mask Display:
      | plot(val(:,1),val(:,2))
      | disp(sys)
      | port_label('input',1,'Address')
      | port_label('input',2,'Value')
      | port_label('output',1,'Result')
      | port_label('output',2,'Error')
  Result : Outport
  Error : Outport  Port=2
  wires:
  S-Function Builder19/1 -> Result/1, Display38/1
  Value/1 -> S-Function Builder19/2
  S-Function Builder19/2 -> Error/1, Display39/1
  Address/1 -> S-Function Builder19/1

== system BEX3_Speed_Contorl_IncrementalEncoders_BLDC_PMSM_2020a/Subsystem1/Enabled Subsystem4/SetEncoderHallCcwOffset ==
  Address : Inport
  Value : Inport  Port=2
  Display84 : Display
      settings: Format=decimal (Stored Integer)
  Display85 : Display
      settings: Format=decimal (Stored Integer)
  S-Function Builder42 : S-Function  Priority=2  FunctionName=SetEncoderHallCcwOffset  SFunctionModules=SetEncoderHallCcwOffset_wrapper  SFunctionDeploymentMode=off  EnableBusSupport=off  mask(S-Function Builder){}
      mask help: Simulink:masks:SFunctionBuilder_MD
      mask init: same as BEX3_Speed_Contorl_IncrementalEncoders_BLDC_PMSM_2020a/Subsystem/Subsystem/S-Function Builder5
      settings: CopyFcn=set_param(gcbh,'LinkStatus','none')  OpenFcn=sfunctionwizard(gcbh)
      mask Display: plot(val(:,1),val(:,2)),disp(sys),port_label('input',1,'Address'),port_label('input',2,'Value'),port_label('output',1,'Result'),port_label('output',2,'Error')
  Result : Outport
  Error : Outport  Port=2
  wires:
  S-Function Builder42/2 -> Error/1, Display85/1
  Value/1 -> S-Function Builder42/2
  S-Function Builder42/1 -> Result/1, Display84/1
  Address/1 -> S-Function Builder42/1

== system BEX3_Speed_Contorl_IncrementalEncoders_BLDC_PMSM_2020a/Subsystem1/Enabled Subsystem5/SetEncoderHallCwOffset ==
  Address : Inport
  Value : Inport  Port=2
  S-Function Builder43 : S-Function  Priority=2  FunctionName=SetEncoderHallCwOffset  SFunctionModules=SetEncoderHallCwOffset_wrapper  SFunctionDeploymentMode=off  EnableBusSupport=off  mask(S-Function Builder){}
      mask help: Simulink:masks:SFunctionBuilder_MD
      mask init: same as BEX3_Speed_Contorl_IncrementalEncoders_BLDC_PMSM_2020a/Subsystem/Subsystem/S-Function Builder5
      settings: CopyFcn=set_param(gcbh,'LinkStatus','none')  OpenFcn=sfunctionwizard(gcbh)
      mask Display:
      | plot(val(:,1),val(:,2))
      | disp(sys)
      | port_label('input',1,'Address')
      | port_label('input',2,'Value')
      | port_label('output',1,'Result')
      | port_label('output',2,'Error')
  Result : Outport
  Error : Outport  Port=2
  wires:
  Address/1 -> S-Function Builder43/1
  S-Function Builder43/2 -> Error/1
  S-Function Builder43/1 -> Result/1
  Value/1 -> S-Function Builder43/2

== system BEX3_Speed_Contorl_IncrementalEncoders_BLDC_PMSM_2020a/Subsystem1/Enabled Subsystem6/SetSpeedLimit ==
  Address : Inport
  Value : Inport  Port=2
  Display40 : Display
      settings: Format=decimal (Stored Integer)
  Display41 : Display
      settings: Format=decimal (Stored Integer)
  S-Function Builder20 : S-Function  Priority=2  FunctionName=SetSpeedLimit  SFunctionModules=SetSpeedLimit_wrapper  SFunctionDeploymentMode=off  EnableBusSupport=off  mask(S-Function Builder){}
      mask help: Simulink:masks:SFunctionBuilder_MD
      mask init: same as BEX3_Speed_Contorl_IncrementalEncoders_BLDC_PMSM_2020a/Subsystem/Subsystem/S-Function Builder5
      settings: CopyFcn=set_param(gcbh,'LinkStatus','none')  OpenFcn=sfunctionwizard(gcbh)
      mask Display:
      | plot(val(:,1),val(:,2))
      | disp(sys)
      | port_label('input',1,'Address')
      | port_label('input',2,'Value')
      | port_label('output',1,'Result')
      | port_label('output',2,'Error')
  Result : Outport
  Error : Outport  Port=2
  wires:
  Value/1 -> S-Function Builder20/2
  S-Function Builder20/1 -> Result/1, Display40/1
  S-Function Builder20/2 -> Error/1, Display41/1
  Address/1 -> S-Function Builder20/1

== system BEX3_Speed_Contorl_IncrementalEncoders_BLDC_PMSM_2020a/Subsystem1/Enabled Subsystem7/SetControlMode ==
  Address : Inport
  Value : Inport  Port=2
  S-Function Builder25 : S-Function  Priority=2  FunctionName=SetControlMode  SFunctionModules=SetControlMode_wrapper  SFunctionDeploymentMode=off  EnableBusSupport=off  mask(S-Function Builder){}
      mask help: Simulink:masks:SFunctionBuilder_MD
      mask init: same as BEX3_Speed_Contorl_IncrementalEncoders_BLDC_PMSM_2020a/Subsystem/Subsystem/S-Function Builder5
      settings: CopyFcn=set_param(gcbh,'LinkStatus','none')  OpenFcn=sfunctionwizard(gcbh)
      mask Display: plot(val(:,1),val(:,2)),disp(sys),port_label('input',1,'Address'),port_label('input',2,'Value'),port_label('output',1,'Result'),port_label('output',2,'Error')
  Result : Outport
  Error : Outport  Port=2
  wires:
  S-Function Builder25/1 -> Result/1
  S-Function Builder25/2 -> Error/1
  Value/1 -> S-Function Builder25/2
  Address/1 -> S-Function Builder25/1

== system BEX3_Speed_Contorl_IncrementalEncoders_BLDC_PMSM_2020a/Subsystem1/Enabled Subsystem8/SetMotorType ==
  Address : Inport
  Value : Inport  Port=2
  Display46 : Display
      settings: Format=decimal (Stored Integer)
  Display47 : Display
      settings: Format=decimal (Stored Integer)
  S-Function Builder23 : S-Function  Priority=2  FunctionName=SetMotorType  SFunctionModules=SetMotorType_wrapper  SFunctionDeploymentMode=off  EnableBusSupport=off  mask(S-Function Builder){}
      mask help: Simulink:masks:SFunctionBuilder_MD
      mask init: same as BEX3_Speed_Contorl_IncrementalEncoders_BLDC_PMSM_2020a/Subsystem/Subsystem/S-Function Builder5
      settings: CopyFcn=set_param(gcbh,'LinkStatus','none')  OpenFcn=sfunctionwizard(gcbh)
      mask Display:
      | plot(val(:,1),val(:,2))
      | disp(sys)
      | port_label('input',1,'Address')
      | port_label('input',2,'Value')
      | port_label('output',1,'Result')
      | port_label('output',2,'Error')
  Result : Outport
  Error : Outport  Port=2
  wires:
  S-Function Builder23/1 -> Result/1, Display46/1
  Value/1 -> S-Function Builder23/2
  S-Function Builder23/2 -> Error/1, Display47/1
  Address/1 -> S-Function Builder23/1

== system BEX3_Speed_Contorl_IncrementalEncoders_BLDC_PMSM_2020a/Subsystem1/Enabled Subsystem9/SetFeedBackControlMode ==
  Address : Inport
  Value : Inport  Port=2
  S-Function Builder21 : S-Function  Priority=2  FunctionName=SetFeedbackControlMode  SFunctionModules=SetFeedbackControlMode_wrapper  SFunctionDeploymentMode=off  EnableBusSupport=off  mask(S-Function Builder){}
      mask help: Simulink:masks:SFunctionBuilder_MD
      mask init: same as BEX3_Speed_Contorl_IncrementalEncoders_BLDC_PMSM_2020a/Subsystem/Subsystem/S-Function Builder5
      settings: CopyFcn=set_param(gcbh,'LinkStatus','none')  OpenFcn=sfunctionwizard(gcbh)
      mask Display:
      | plot(val(:,1),val(:,2))
      | disp(sys)
      | port_label('input',1,'Address')
      | port_label('input',2,'Value')
      | port_label('output',1,'Result')
      | port_label('output',2,'Error')
  Result : Outport
  Error : Outport  Port=2
  wires:
  S-Function Builder21/1 -> Result/1
  S-Function Builder21/2 -> Error/1
  Value/1 -> S-Function Builder21/2
  Address/1 -> S-Function Builder21/1

== system BEX3_Speed_Contorl_IncrementalEncoders_BLDC_PMSM_2020a/Subsystem4/Subsystem1/GetPositionCountsFeedback ==
  Address : Inport
  S-Function Builder73 : S-Function  Priority=3  FunctionName=GetPositionCountsFeedback  SFunctionModules=GetPositionCountsFeedback_wrapper  SFunctionDeploymentMode=off  EnableBusSupport=off  mask(S-Function Builder){}
      mask help: Simulink:masks:SFunctionBuilder_MD
      mask init: same as BEX3_Speed_Contorl_IncrementalEncoders_BLDC_PMSM_2020a/Subsystem/Subsystem/S-Function Builder5
      settings: CopyFcn=set_param(gcbh,'LinkStatus','none')  OpenFcn=sfunctionwizard(gcbh)
      mask Display: plot(val(:,1),val(:,2)),disp(sys),port_label('input',1,'Address'),port_label('output',1,'Result'),port_label('output',2,'Error')
  Result : Outport
  Error : Outport  Port=2
  wires:
  Address/1 -> S-Function Builder73/1
  S-Function Builder73/2 -> Error/1
  S-Function Builder73/1 -> Result/1

== system BEX3_Speed_Contorl_IncrementalEncoders_BLDC_PMSM_2020a/Subsystem4/Subsystem2/GetSpeedFeedback ==
  Address : Inport
  S-Function Builder66 : S-Function  Priority=3  FunctionName=GetSpeedFeedback  SFunctionModules=GetSpeedFeedback_wrapper  SFunctionDeploymentMode=off  EnableBusSupport=off  mask(S-Function Builder){}
      mask help: Simulink:masks:SFunctionBuilder_MD
      mask init: same as BEX3_Speed_Contorl_IncrementalEncoders_BLDC_PMSM_2020a/Subsystem/Subsystem/S-Function Builder5
      settings: CopyFcn=set_param(gcbh,'LinkStatus','none')  OpenFcn=sfunctionwizard(gcbh)
      mask Display: plot(val(:,1),val(:,2)),disp(sys),port_label('input',1,'Address'),port_label('output',1,'Result'),port_label('output',2,'Error')
  Result : Outport
  Error : Outport  Port=2
  wires:
  Address/1 -> S-Function Builder66/1
  S-Function Builder66/1 -> Result/1
  S-Function Builder66/2 -> Error/1

== system BEX3_Speed_Contorl_IncrementalEncoders_BLDC_PMSM_2020a/Subsystem4/Subsystem3/GetQuadratureCurrentIqFeedback ==
  Address : Inport
  S-Function Builder57 : S-Function  Priority=3  FunctionName=GetQuadratureCurrentIqFeedback  SFunctionModules=GetQuadratureCurrentIqFeedback_wrapper  SFunctionDeploymentMode=off  EnableBusSupport=off  mask(S-Function Builder){}
      mask help: Simulink:masks:SFunctionBuilder_MD
      mask init: same as BEX3_Speed_Contorl_IncrementalEncoders_BLDC_PMSM_2020a/Subsystem/Subsystem/S-Function Builder5
      settings: CopyFcn=set_param(gcbh,'LinkStatus','none')  OpenFcn=sfunctionwizard(gcbh)
      mask Display: plot(val(:,1),val(:,2)),disp(sys),port_label('input',1,'Address'),port_label('output',1,'Result'),port_label('output',2,'Error')
  Result : Outport
  Error : Outport  Port=2
  wires:
  S-Function Builder57/2 -> Error/1
  Address/1 -> S-Function Builder57/1
  S-Function Builder57/1 -> Result/1

== system BEX3_Speed_Contorl_IncrementalEncoders_BLDC_PMSM_2020a/Tx/Subsystem1/Enabled Subsystem ==
  TorqueRef : Inport
  Enable : EnablePort
  Constant : Constant  Value=0  OutDataTypeStr=Inherit: Inherit via back propagation
  SetTorqueReferenceIq : Subsystem
  Result : Outport
  Error : Outport  Port=2
  wires:
  Constant/1 -> SetTorqueReferenceIq/1(Address)
  TorqueRef/1 -> SetTorqueReferenceIq/2(Value)
  SetTorqueReferenceIq/1(Result) -> Result/1
  SetTorqueReferenceIq/2(Error) -> Error/1

== system BEX3_Speed_Contorl_IncrementalEncoders_BLDC_PMSM_2020a/Tx/Subsystem1/Enabled Subsystem1 ==
  Speed : Inport
  Enable : EnablePort
  Constant : Constant  Value=0  OutDataTypeStr=Inherit: Inherit via back propagation
  SpeedRef : Subsystem
  Result : Outport
  Error : Outport  Port=2
  wires:
  Constant/1 -> SpeedRef/1(Address)
  Speed/1 -> SpeedRef/2(Value)
  SpeedRef/2(Error) -> Error/1
  SpeedRef/1(Result) -> Result/1

== system BEX3_Speed_Contorl_IncrementalEncoders_BLDC_PMSM_2020a/Tx/Subsystem1/Enabled Subsystem10 ==
  EmergencyStop : Inport
  Enable : EnablePort
  Data Type Conversion : DataTypeConversion
  EmergencyStop1 : Subsystem
  Result : Outport
  Error : Outport  Port=2
  wires:
  EmergencyStop/1 -> Data Type Conversion/1
  EmergencyStop1/2(Error) -> Error/1
  EmergencyStop1/1(Result) -> Result/1
  Data Type Conversion/1 -> EmergencyStop1/1(Address)

== system BEX3_Speed_Contorl_IncrementalEncoders_BLDC_PMSM_2020a/Tx/Subsystem1/Enabled Subsystem2 ==
  PositionRef : Inport
  Enable : EnablePort
  Constant : Constant  Value=0  OutDataTypeStr=Inherit: Inherit via back propagation
  SetPositionRef : Subsystem
  Result : Outport
  Error : Outport  Port=2
  wires:
  PositionRef/1 -> SetPositionRef/2(Value)
  Constant/1 -> SetPositionRef/1(Address)
  SetPositionRef/2(Error) -> Error/1
  SetPositionRef/1(Result) -> Result/1

== system BEX3_Speed_Contorl_IncrementalEncoders_BLDC_PMSM_2020a/Tx/Subsystem1/Enabled Subsystem3 ==
  Direction : Inport
  Enable : EnablePort
  Constant : Constant  Value=0  OutDataTypeStr=Inherit: Inherit via back propagation
  SetMotorDirection : Subsystem
  Result : Outport
  Error : Outport  Port=2
  wires:
  Constant/1 -> SetMotorDirection/1(Address)
  Direction/1 -> SetMotorDirection/2(Value)
  SetMotorDirection/2(Error) -> Error/1
  SetMotorDirection/1(Result) -> Result/1

== system BEX3_Speed_Contorl_IncrementalEncoders_BLDC_PMSM_2020a/Tx/Subsystem1/Enabled Subsystem4 ==
  SpeedKp : Inport
  Enable : EnablePort
  Constant26 : Constant  Value=0  OutDataTypeStr=uint8
  SetSpeed Kp : Subsystem
  Result : Outport
  Error : Outport  Port=2
  wires:
  SetSpeed Kp/2(Error) -> Error/1
  SetSpeed Kp/1(Result) -> Result/1
  Constant26/1 -> SetSpeed Kp/1(Address)
  SpeedKp/1 -> SetSpeed Kp/2(Value)

== system BEX3_Speed_Contorl_IncrementalEncoders_BLDC_PMSM_2020a/Tx/Subsystem1/Enabled Subsystem5 ==
  SpeedKi : Inport
  Enable : EnablePort
  Constant28 : Constant  Value=0  OutDataTypeStr=uint8
  SetSpeed Ki : Subsystem
  Result : Outport
  Error : Outport  Port=2
  wires:
  Constant28/1 -> SetSpeed Ki/1(Address)
  SpeedKi/1 -> SetSpeed Ki/2(Value)
  SetSpeed Ki/2(Error) -> Error/1
  SetSpeed Ki/1(Result) -> Result/1

== system BEX3_Speed_Contorl_IncrementalEncoders_BLDC_PMSM_2020a/Tx/Subsystem1/Enabled Subsystem6 ==
  PositionKp : Inport
  Enable : EnablePort
  Constant60 : Constant  Value=0  OutDataTypeStr=uint8
  SetPositionControllerKp : Subsystem
  Result : Outport
  Error : Outport  Port=2
  wires:
  PositionKp/1 -> SetPositionControllerKp/2(Value)
  SetPositionControllerKp/2(Error) -> Error/1
  SetPositionControllerKp/1(Result) -> Result/1
  Constant60/1 -> SetPositionControllerKp/1(Address)

== system BEX3_Speed_Contorl_IncrementalEncoders_BLDC_PMSM_2020a/Tx/Subsystem1/Enabled Subsystem7 ==
  PositionKi : Inport
  Enable : EnablePort
  Constant62 : Constant  Value=0  OutDataTypeStr=uint8
  SetPositionControllerKi : Subsystem
  Result : Outport
  Error : Outport  Port=2
  wires:
  PositionKi/1 -> SetPositionControllerKi/2(Value)
  SetPositionControllerKi/2(Error) -> Error/1
  SetPositionControllerKi/1(Result) -> Result/1
  Constant62/1 -> SetPositionControllerKi/1(Address)

== system BEX3_Speed_Contorl_IncrementalEncoders_BLDC_PMSM_2020a/Tx/Subsystem1/Enabled Subsystem8 ==
  CurrentKp : Inport
  Enable : EnablePort
  Constant50 : Constant  Value=0  OutDataTypeStr=uint8
  SetCurrentControlKp : Subsystem
  Result : Outport
  Error : Outport  Port=2
  wires:
  CurrentKp/1 -> SetCurrentControlKp/2(Value)
  SetCurrentControlKp/2(Error) -> Error/1
  SetCurrentControlKp/1(Result) -> Result/1
  Constant50/1 -> SetCurrentControlKp/1(Address)

== system BEX3_Speed_Contorl_IncrementalEncoders_BLDC_PMSM_2020a/Tx/Subsystem1/Enabled Subsystem9 ==
  CurrentKi : Inport
  Enable : EnablePort
  Constant52 : Constant  Value=0  OutDataTypeStr=uint8
  SetCurrentControlKi : Subsystem
  Result : Outport
  Error : Outport  Port=2
  wires:
  CurrentKi/1 -> SetCurrentControlKi/2(Value)
  SetCurrentControlKi/2(Error) -> Error/1
  SetCurrentControlKi/1(Result) -> Result/1
  Constant52/1 -> SetCurrentControlKi/1(Address)

== system BEX3_Speed_Contorl_IncrementalEncoders_BLDC_PMSM_2020a/Tx/Subsystem1/Enabled Subsystem/SetTorqueReferenceIq ==
  Address : Inport  OutDataTypeStr=uint8  LockScale=on
  Value : Inport  Port=2  OutDataTypeStr=single  LockScale=on
  Display12 : Display
      settings: Format=decimal (Stored Integer)
  Display13 : Display
      settings: Format=decimal (Stored Integer)
  S-Function Builder4 : S-Function  Priority=2  FunctionName=SetTorqueReferenceIq  SFunctionModules=SetTorqueReferenceIq_wrapper  SFunctionDeploymentMode=off  EnableBusSupport=off  mask(S-Function Builder){}
      mask help: Simulink:masks:SFunctionBuilder_MD
      mask init: same as BEX3_Speed_Contorl_IncrementalEncoders_BLDC_PMSM_2020a/Subsystem/Subsystem/S-Function Builder5
      settings: CopyFcn=set_param(gcbh,'LinkStatus','none')  OpenFcn=sfunctionwizard(gcbh)
      mask Display: plot(val(:,1),val(:,2)),disp(sys),port_label('input',1,'Address'),port_label('input',2,'Value'),port_label('output',1,'Result'),port_label('output',2,'Error')
  Result : Outport  OutDataTypeStr=boolean
  Error : Outport  Port=2  OutDataTypeStr=int32
  wires:
  Address/1 -> S-Function Builder4/1
  S-Function Builder4/2 -> Error/1, Display13/1
  S-Function Builder4/1 -> Result/1, Display12/1
  Value/1 -> S-Function Builder4/2
